simulink model "reichardt_array_EMD"  (Simulink 9.3)
settings: Solver=ode45  StartTime=0.0  StopTime=setStopTime  FixedStep=0.0005  RelTol=1e-3  EnableMultiTasking=on
model workspace (MAT data in the model file):
  bodyAmp = 0
  bodyPhase = 0
  freq = 628.318530718
  headAmp = 0
  headPhase = 0
  imageData = [0.00303351691359 0.00909998476947 0.0151647548087 0.0212266954775 0.0272846757084 0.0333375651143 0.0393842341832 0.0454235544723 0.0514543988027 0.0574756414532 0.0634861583552 0.0694848272865 ... (8204 elements, 1x8204)]
  outputTimeList = [1 1.0001 1.0002 1.0003 1.0004 1.0005 1.0006 1.0007 1.0008 1.0009 1.001 1.0011 1.0012 1.0013 1.0014 1.0015 1.0016 1.0017 1.0018 1.0019 1.002 1.0021 1.0022 1.0023 1.0024 1.0025 1.0026 1.0027 1.0028 1.0029 1.003 1.0031 1.0032 1.0033 1.0034 1.0035 1.0036 1.0037 1.0038 1.0039 1.004 1.0041 1.0042 1.0043 1.0044 1.0045 1.0046 1.0047 1.0048 1.0049 1.005 1.0051 1.0052 1.0053 1.0054 1.0055 1.0056 1.0057 1.0058 1.0059 1.006 1.0061 1.0062 1.0063 1.0064 1.0065 1.0066 1.0067 1.0068 1.0069 1.007 1.0071 1.0072 1.0073 1.0074 1.0075 1.0076 1.0077 1.0078 1.0079 1.008 1.0081 1.0082 1.0083 1.0084 1.0085 1.0086 1.0087 1.0088 1.0089 1.009 1.0091 1.0092 1.0093 1.0094 1.0095 1.0096 1.0097 1.0098 1.0099 1.01]
  setStopTime = 1.01
  stimAmp = 5
  temporalFilt = 0.046
  timeConstant = 0.046
values from neighbouring files (symbols this model uses):
  timeConstant = 46-3    (= 43)    [TEST.m]
libraries: visionsources x1
settings Model: LogicAnalyzerSignalOrdering=a71c693a-e045-49f2-9a2b-fd1d6fda7f8e,94723d94-0fb9-48a1-a8be-bee64210528d,ca6ec58f-53b8-4cb0-954b-e32596e728e1,6b902a21-b312-494c-94da-f4c8e853617c,db28250c-7404-4e50-ae35-76410c95bf8e,836d504f-1a60-4509-b72a-a4806fe259f8,c3d22241-23bf-4d79-9aab-67dc7151a41f  Creator=Shane  LastModifiedBy=BC  SimulationMode=accelerator
settings DataIOCC: SignalLoggingSaveFormat=Dataset  ReturnWorkspaceOutputs=on  OutputOption=SpecifiedOutputTimes  OutputTimes=outputTimeList
settings OptimizationCC: ExpressionDepthLimit=2147483647  EfficientMapNaN2IntZero=off  LifeSpan=auto  SimCompilerOptimization=on
settings DebuggingCC: StateNameClashWarn=warning
settings HardwareCC: TargetBitPerPointer=64  TargetBitPerSizeT=64  TargetBitPerPtrDiffT=64  TargetLongLongMode=on  TargetIntDivRoundTo=Zero  TargetEndianess=LittleEndian  TargetWordSize=64  TargetHWDeviceType=MATLAB Host  ProdEqTarget=off
settings RTWCC: SystemTargetFile=accel.tlc  TemplateMakefile=accel_default_tmf  RTWVerbose=off  RTWUseLocalCustomCode=on
settings CodeAppCC: MaxIdLength=128  StateflowObjectComments=off
settings STFCustomTargetCC: ConcurrentExecutionCompliant=on  MATLABClassNameForMDSCustomization=Simulink.SoftwareTarget.TargetSpecificTriggerConfigurationBase  SystemTargetFile=accel.tlc

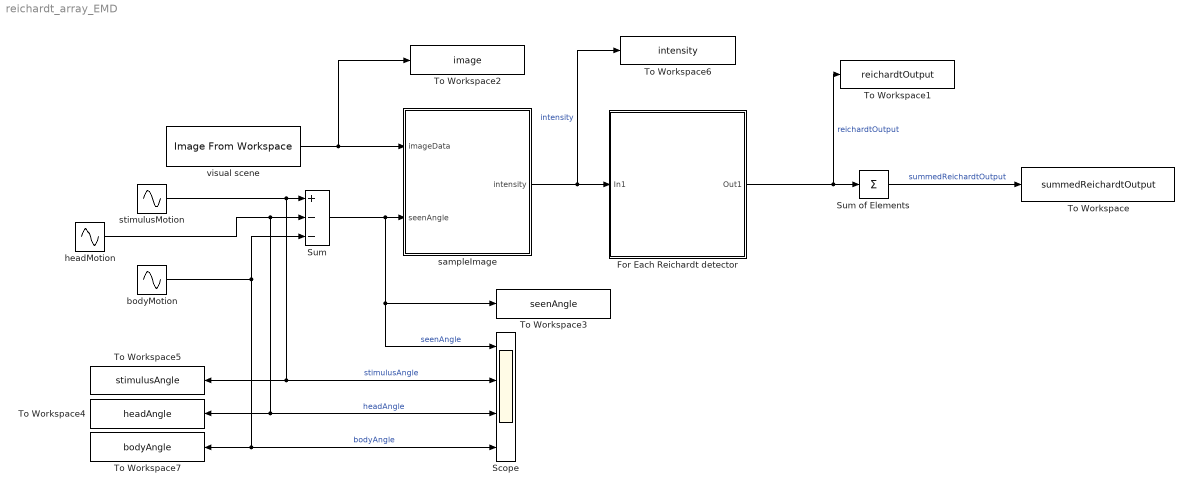
== system reichardt_array_EMD ==
  For Each Reichardt detector : Subsystem  TreatAsAtomicUnit=on
  Scope : Scope  NumInputPorts=4
  Sum : Sum  Inputs=+--
  Sum of Elements : Sum  Inputs=+
  To Workspace : ToWorkspace  VariableName=summedReichardtOutput  SaveFormat=Timeseries  SampleTime=-1
  To Workspace1 : ToWorkspace  VariableName=reichardtOutput  SaveFormat=Timeseries  SampleTime=-1
  To Workspace2 : ToWorkspace  VariableName=image  SaveFormat=Timeseries  SampleTime=-1
  To Workspace3 : ToWorkspace  VariableName=seenAngle  SaveFormat=Timeseries  SampleTime=-1
  To Workspace4 : ToWorkspace  VariableName=headAngle  SaveFormat=Timeseries  SampleTime=-1
  To Workspace5 : ToWorkspace  VariableName=stimulusAngle  SaveFormat=Timeseries  SampleTime=-1
  To Workspace6 : ToWorkspace  VariableName=intensity  SaveFormat=Timeseries  SampleTime=-1
  To Workspace7 : ToWorkspace  VariableName=bodyAngle  SaveFormat=Timeseries  SampleTime=-1
  bodyMotion : Sin  Amplitude=bodyAmp  Frequency=freq  Phase=bodyPhase  SampleTime=0
  headMotion : Sin  Amplitude=headAmp  Frequency=freq  Phase=headPhase  SampleTime=0
  sampleImage : MATLAB Function  TreatAsAtomicUnit=on
  stimulusMotion : Sin  Amplitude=stimAmp  Frequency=freq  SampleTime=0
  visual scene : visionsources/Image From Workspace  Tag=vipblks_nd  ImageValue=imageData  Ts=inf  imagePorts=One multidimensional signal  OutPortLabels=R|G|B  ImageDataType=double  Signed=on  WordLength=16  sdImageDataType=sfix(16)  FractionLengthMode=User-defined  FractionLength=15
      settings: SourceProductName=Computer Vision Toolbox  SourceProductBaseCode=VP
  wires:
  For Each Reichardt detector/1(Out1) -> To Workspace1/1, Sum of Elements/1  "reichardtOutput"
  Sum of Elements/1 -> To Workspace/1  "summedReichardtOutput"
  sampleImage/1(intensity) -> To Workspace6/1, For Each Reichardt detector/1(In1)  "intensity"
  visual scene/1 -> To Workspace2/1, sampleImage/1(imageData)
  stimulusMotion/1 -> To Workspace5/1, Scope/2, Sum/1  "stimulusAngle"
  headMotion/1 -> To Workspace4/1, Scope/3, Sum/2  "headAngle"
  Sum/1 -> Scope/1, To Workspace3/1, sampleImage/2(seenAngle)  "seenAngle"
  bodyMotion/1 -> Sum/3, To Workspace7/1, Scope/4  "bodyAngle"

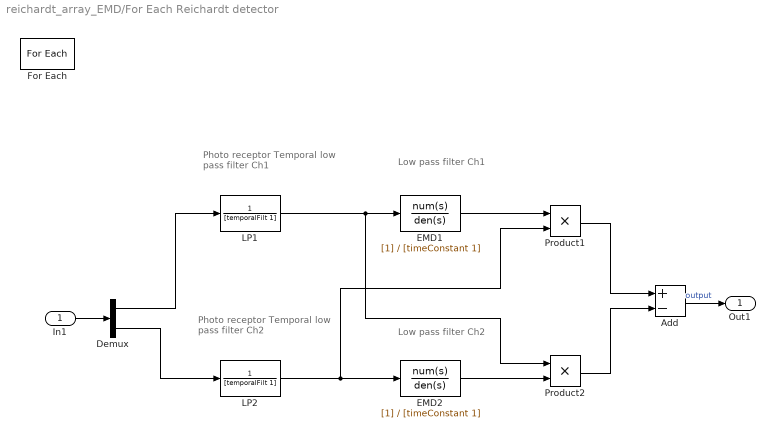
== system reichardt_array_EMD/For Each Reichardt detector ==
  note: Photo receptor
      | Temporal low pass filter
      | Ch2
  note: Photo receptor
      | Temporal low pass filter
      | Ch1
  note: Low pass filter
      | Ch1
  note: Low pass filter
      | Ch2
  In1 : Inport  Partition=on  PartitionDimension=1  PartitionWidth=1  PartitionOffset=0
  Add : Sum  Inputs=+-
  Demux : Demux  Outputs=2
  EMD1 : TransferFcn  Denominator=[timeConstant 1]
  EMD2 : TransferFcn  Denominator=[timeConstant 1]
  For Each : ForEach  DisableCoverage=on  IndexMode=One-based
  LP1 : TransferFcn  Numerator=1  Denominator=[temporalFilt 1]
  LP2 : TransferFcn  Numerator=1  Denominator=[temporalFilt 1]
  Product1 : Product  RndMeth=Zero
  Product2 : Product  RndMeth=Zero
  Out1 : Outport  ConcatenationDimension=1
  wires:
  EMD1/1 -> Product1/1
  Product1/1 -> Add/1
  Product2/1 -> Add/2
  EMD2/1 -> Product2/2
  Add/1 -> Out1/1  "output"
  Demux/1 -> LP1/1
  In1/1 -> Demux/1
  Demux/2 -> LP2/1
  LP2/1 -> EMD2/1, Product1/2
  LP1/1 -> EMD1/1, Product2/1

== matlab function sampleImage ==
  data: imageData input double; intensity output double size=360,2; seenAngle input double
function intensity = fcn(imageData,seenAngle)
%#codegen

imageWidth = length(imageData);

% Subsample with resolution of compound eye
sampleCoord = 0:359;
sampleCoord = sampleCoord + seenAngle;
sampleCoord = mod(sampleCoord,360);
temp        = interp1(linspace(0,360,imageWidth),imageData,sampleCoord);

% Create output signals
intensity = [temp(:), circshift(temp(:),-1)];
